simulink model "gm_sd_filter_tb"  (R2022b)
settings: Solver=VariableStepAuto  StartTime=0.0  StopTime=t_stop  RelTol=1e-3
undefined symbols (not defined in the file or in its folder): bitwidths, ts
settings Model: Creator=Legion  LastModifiedBy=qaztr
settings SolverCC: AlgebraicLoopSolver=TrustRegion
settings OptimizationCC: BlockReduction=off  ConditionallyExecuteInputs=off
settings DebuggingCC: InheritedTsInSrcMsg=none  UnconnectedInputMsg=warning  UnconnectedOutputMsg=warning  UnconnectedLineMsg=warning  SFMachineParentedDataDiag=warning
settings ModelReferenceCC: EnableRefExpFcnMdlSchedulingChecks=on
settings RTWCC: DLArmComputeVersion=19.05

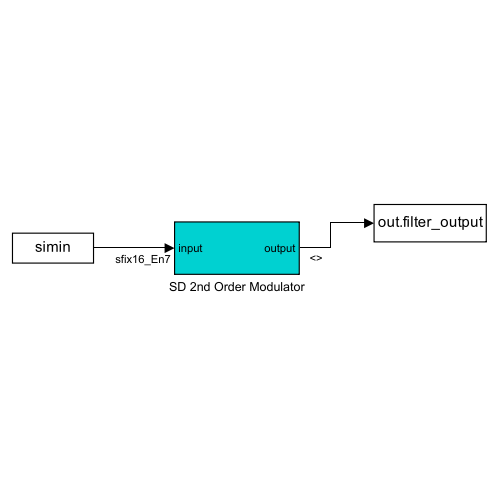
[thumbnail: Simulink's stored preview of the top-level diagram]
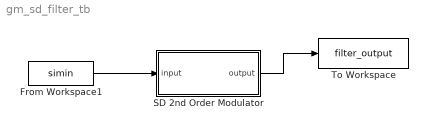
== system gm_sd_filter_tb ==
  From Workspace1 : FromWorkspace  VariableName=simin  SampleTime=ts  Interpolate=off  OutputAfterFinalValue=Holding final value
  SD 2nd Order Modulator : Subsystem
  To Workspace : ToWorkspace  VariableName=filter_output  SaveFormat=Structure With Time  SampleTime=-1
  wires:
  From Workspace1/1 -> SD 2nd Order Modulator/1(input)
  SD 2nd Order Modulator/1(output) -> To Workspace/1

== system gm_sd_filter_tb/SD 2nd Order Modulator ==
  input : Inport  OutDataTypeStr=fixdt(1, 16, 7)  PortDimensions=1  SampleTime=8.85770975056689e-08
  SD 2nd Order Modulator : Subsystem
  SD 2nd Order Modulator1 : Subsystem
  SD Filter : Subsystem
  output : Outport  SampleTime=8.85770975056689e-08
  wires:
  input/1 -> SD 2nd Order Modulator1/1(in)
  SD 2nd Order Modulator/1(out) -> output/1, SD Filter/2(feedback)
  SD 2nd Order Modulator1/1(out) -> SD Filter/1(input)
  SD Filter/1(output) -> SD 2nd Order Modulator/1(in)

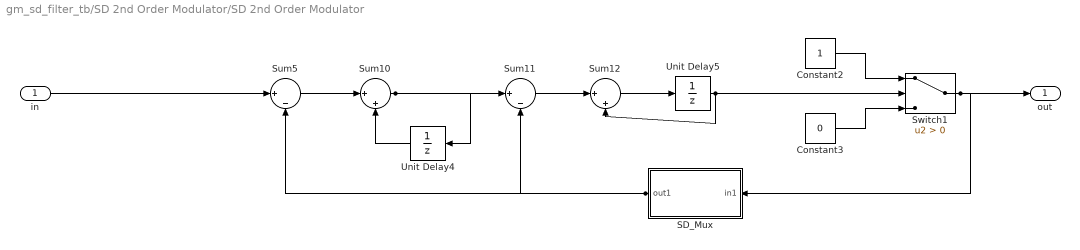
== system gm_sd_filter_tb/SD 2nd Order Modulator/SD 2nd Order Modulator ==
  in : Inport  OutDataTypeStr=fixdt(1, 47, 22)  PortDimensions=1  SampleTime=8.85770975056689e-08
  Constant2 : Constant  OutDataTypeStr=boolean
  Constant3 : Constant  Value=0  OutDataTypeStr=boolean
  SD_Mux : Subsystem  mask{a=fi(0,1,16,7,"hex","0080"), Parameter2=fixdt(1,32,23)}
      mask prompts: a "Amp"; Parameter2 "Data Type"
  Sum10 : Sum  Inputs=||+|+  OutDataTypeStr=Inherit: Same as accumulator
  Sum11 : Sum  Inputs=||+|-  OutDataTypeStr=Inherit: Same as accumulator
  Sum12 : Sum  Inputs=||+|+  OutDataTypeStr=Inherit: Same as accumulator
  Sum5 : Sum  Inputs=||+|-  OutDataTypeStr=Inherit: Same as accumulator
  Switch1 : Switch  Criteria=u2 > Threshold  SaturateOnIntegerOverflow=off  InputSameDT=off
  Unit Delay4 : UnitDelay  SampleTime=-1  HasFrameUpgradeWarning=on
  Unit Delay5 : UnitDelay  SampleTime=-1  HasFrameUpgradeWarning=on
  out : Outport  SampleTime=8.85770975056689e-08
  wires:
  in/1 -> Sum5/1
  Constant2/1 -> Switch1/1
  Constant3/1 -> Switch1/3
  SD_Mux/1(out1) -> Sum5/2, Sum11/2
  Sum10/1 -> Sum11/1, Unit Delay4/1
  Sum11/1 -> Sum12/1
  Sum12/1 -> Unit Delay5/1
  Sum5/1 -> Sum10/1
  Switch1/1 -> SD_Mux/1(in1), out/1
  Unit Delay4/1 -> Sum10/2
  Unit Delay5/1 -> Switch1/2, Sum12/2

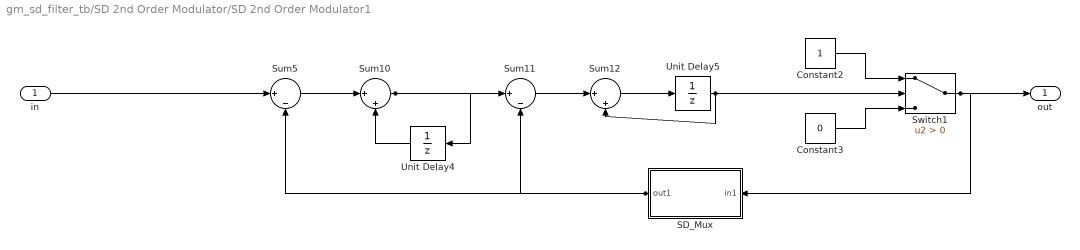
== system gm_sd_filter_tb/SD 2nd Order Modulator/SD 2nd Order Modulator1 ==
  in : Inport  OutDataTypeStr=fixdt(1, 16, 7)  PortDimensions=1  SampleTime=8.85770975056689e-08
  Constant2 : Constant  OutDataTypeStr=boolean
  Constant3 : Constant  Value=0  OutDataTypeStr=boolean
  SD_Mux : Subsystem  mask{a=fi(0,1,16,7,"hex","0080"), Parameter2=fixdt(1,32,23)}
      mask prompts: a "Amp"; Parameter2 "Data Type"
  Sum10 : Sum  Inputs=||+|+  OutDataTypeStr=Inherit: Same as accumulator
  Sum11 : Sum  Inputs=||+|-  OutDataTypeStr=Inherit: Same as accumulator
  Sum12 : Sum  Inputs=||+|+  OutDataTypeStr=Inherit: Same as accumulator
  Sum5 : Sum  Inputs=||+|-  OutDataTypeStr=Inherit: Same as accumulator
  Switch1 : Switch  Criteria=u2 > Threshold  SaturateOnIntegerOverflow=off  InputSameDT=off
  Unit Delay4 : UnitDelay  SampleTime=-1  HasFrameUpgradeWarning=on
  Unit Delay5 : UnitDelay  SampleTime=-1  HasFrameUpgradeWarning=on
  out : Outport  SampleTime=8.85770975056689e-08
  wires:
  in/1 -> Sum5/1
  Constant2/1 -> Switch1/1
  Constant3/1 -> Switch1/3
  SD_Mux/1(out1) -> Sum5/2, Sum11/2
  Sum10/1 -> Sum11/1, Unit Delay4/1
  Sum11/1 -> Sum12/1
  Sum12/1 -> Unit Delay5/1
  Sum5/1 -> Sum10/1
  Switch1/1 -> SD_Mux/1(in1), out/1
  Unit Delay4/1 -> Sum10/2
  Unit Delay5/1 -> Switch1/2, Sum12/2

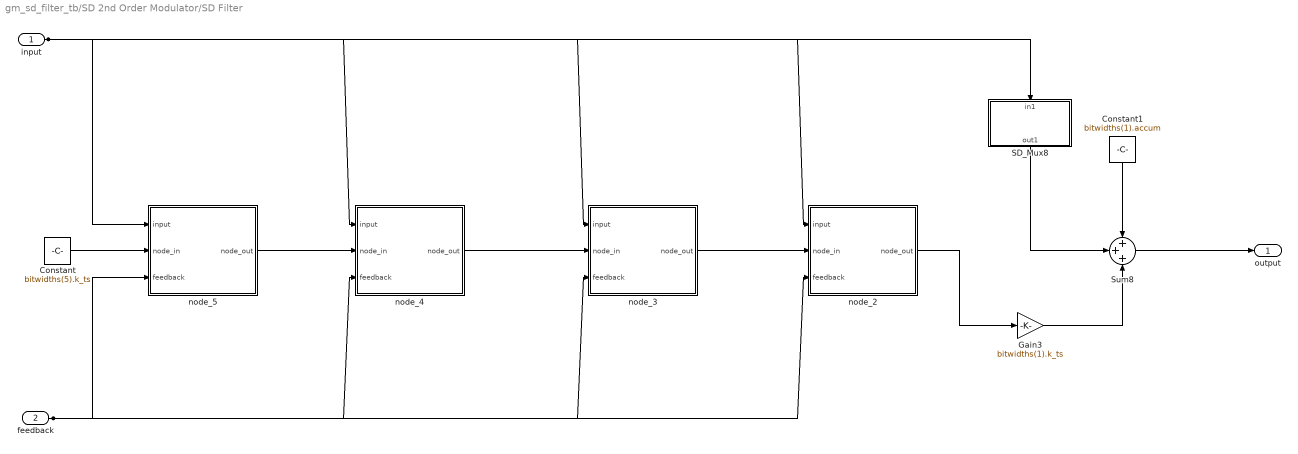
== system gm_sd_filter_tb/SD 2nd Order Modulator/SD Filter ==
  input : Inport  OutDataTypeStr=boolean  PortDimensions=1  SampleTime=8.85770975056689e-08
  feedback : Inport  Port=2  OutDataTypeStr=boolean  PortDimensions=1  SampleTime=8.85770975056689e-08
  Constant : Constant  Value=bitwidths(5).k_ts
  Constant1 : Constant  Value=bitwidths(1).accum
  Gain3 : Gain  Gain=bitwidths(1).k_ts  RndMeth=Round
  SD_Mux8 : Subsystem  mask{a=fi(0,1,24,22,"hex","001062"), Parameter2=Inherit: Inherit via internal rule}
      mask prompts: a "Amp"; Parameter2 "Data Type"
  Sum8 : Sum  Inputs=+++  OutDataTypeStr=Inherit: Same as accumulator
  node_2 : Subsystem  mask{Parameter1=fi(0,1,21,8,"hex","064305"), Parameter2=fi(0,1,21,8,"hex","00000c"), Parameter3=fi(0,1,12,11,"hex","001"), Parameter4=fi(0,1,33,8,"hex","000000000")}
      mask prompts: Parameter1 "alpha"; Parameter2 "beta"; Parameter3 "k"; Parameter4 "Accumulator"
  node_3 : Subsystem  mask{Parameter1=fi(0,1,25,8,"hex","04b7082"), Parameter2=fi(0,1,25,8,"hex","000adcd"), Parameter3=fi(0,1,12,11,"hex","001"), Parameter4=fi(0,1,33,8,"hex","000000000")}
      mask prompts: Parameter1 "alpha"; Parameter2 "beta"; Parameter3 "k"; Parameter4 "Accumulator"
  node_4 : Subsystem  mask{Parameter1=fi(0,1,21,8,"hex","07523c"), Parameter2=fi(0,1,21,8,"hex","0022af"), Parameter3=fi(0,1,12,11,"hex","001"), Parameter4=fi(0,1,33,8,"hex","000000000")}
      mask prompts: Parameter1 "alpha"; Parameter2 "beta"; Parameter3 "k"; Parameter4 "Accumulator"
  node_5 : Subsystem  mask{Parameter1=fi(0,1,16,0,"hex","2bbf"), Parameter2=fi(0,1,16,0,"hex","000b"), Parameter3=fi(0,1,2,1,"hex","0"), Parameter4=fi(0,1,25,0,"hex","0000000")}
      mask prompts: Parameter1 "alpha"; Parameter2 "beta"; Parameter3 "k"; Parameter4 "Accumulator"
  output : Outport  SampleTime=8.85770975056689e-08
  wires:
  input/1 -> node_5/1(input), node_4/1(input), node_3/1(input), node_2/1(input), SD_Mux8/1(in1)
  feedback/1 -> node_5/3(feedback), node_4/3(feedback), node_2/3(feedback), node_3/3(feedback)
  Constant/1 -> node_5/2(node_in)
  Constant1/1 -> Sum8/1
  Gain3/1 -> Sum8/3
  SD_Mux8/1(out1) -> Sum8/2
  Sum8/1 -> output/1
  node_2/1(node_out) -> Gain3/1
  node_3/1(node_out) -> node_2/2(node_in)
  node_4/1(node_out) -> node_3/2(node_in)
  node_5/1(node_out) -> node_4/2(node_in)

== system gm_sd_filter_tb/SD 2nd Order Modulator/SD 2nd Order Modulator/SD_Mux ==
  in1 : Inport  OutDataTypeStr=boolean  PortDimensions=1  SampleTime=8.85770975056689e-08
  Constant2 : Constant  Value=a
  Constant3 : Constant  Value=-a
  Switch1 : Switch  Criteria=u2 > Threshold  SaturateOnIntegerOverflow=off  InputSameDT=off
  out1 : Outport  SampleTime=8.85770975056689e-08
  wires:
  in1/1 -> Switch1/2
  Constant2/1 -> Switch1/1
  Constant3/1 -> Switch1/3
  Switch1/1 -> out1/1

== system gm_sd_filter_tb/SD 2nd Order Modulator/SD 2nd Order Modulator1/SD_Mux ==
  in1 : Inport  OutDataTypeStr=boolean  PortDimensions=1  SampleTime=8.85770975056689e-08
  Constant2 : Constant  Value=a
  Constant3 : Constant  Value=-a
  Switch1 : Switch  Criteria=u2 > Threshold  SaturateOnIntegerOverflow=off  InputSameDT=off
  out1 : Outport  SampleTime=8.85770975056689e-08
  wires:
  in1/1 -> Switch1/2
  Constant2/1 -> Switch1/1
  Constant3/1 -> Switch1/3
  Switch1/1 -> out1/1

== system gm_sd_filter_tb/SD 2nd Order Modulator/SD Filter/SD_Mux8 ==
  in1 : Inport  OutDataTypeStr=boolean  PortDimensions=1  SampleTime=8.85770975056689e-08
  Constant2 : Constant  Value=a
  Constant3 : Constant  Value=-a
  Switch1 : Switch  Criteria=u2 > Threshold  SaturateOnIntegerOverflow=off  InputSameDT=off
  out1 : Outport  SampleTime=8.85770975056689e-08
  wires:
  in1/1 -> Switch1/2
  Constant2/1 -> Switch1/1
  Constant3/1 -> Switch1/3
  Switch1/1 -> out1/1

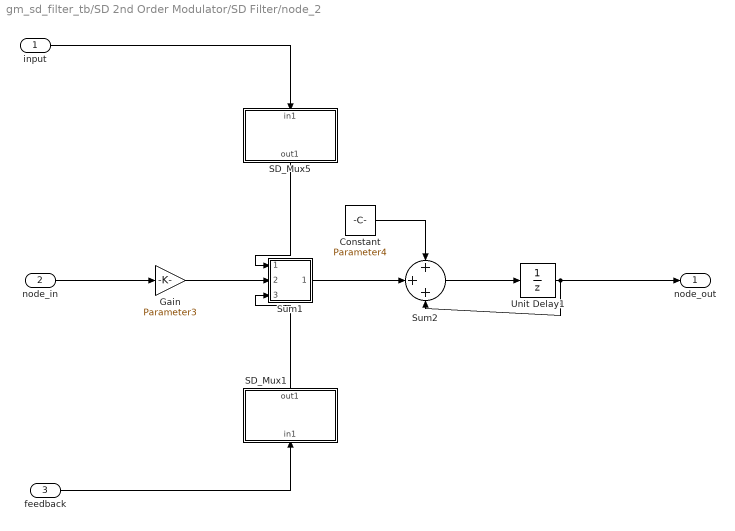
== system gm_sd_filter_tb/SD 2nd Order Modulator/SD Filter/node_2 ==
  input : Inport  OutDataTypeStr=boolean  PortDimensions=1  SampleTime=8.85770975056689e-08
  node_in : Inport  Port=2  OutDataTypeStr=fixdt(1, 33, 8)  PortDimensions=1  SampleTime=8.85770975056689e-08
  feedback : Inport  Port=3  OutDataTypeStr=boolean  PortDimensions=1  SampleTime=8.85770975056689e-08
  Constant : Constant  Value=Parameter4
  Gain : Gain  Gain=Parameter3  RndMeth=Round
  SD_Mux1 : Subsystem  mask{a=fi(0,1,21,8,"hex","064305"), Parameter2=Inherit: Inherit via internal rule}
      mask prompts: a "Amp"; Parameter2 "Data Type"
  SD_Mux5 : Subsystem  mask{a=fi(0,1,21,8,"hex","00000c"), Parameter2=Inherit: Inherit via internal rule}
      mask prompts: a "Amp"; Parameter2 "Data Type"
  Sum1 : Subsystem
  Sum2 : Sum  Inputs=+++  OutDataTypeStr=Inherit: Same as accumulator
  Unit Delay1 : UnitDelay  SampleTime=-1  HasFrameUpgradeWarning=on
  node_out : Outport  SampleTime=8.85770975056689e-08
  wires:
  input/1 -> SD_Mux5/1(in1)
  node_in/1 -> Gain/1
  feedback/1 -> SD_Mux1/1(in1)
  Constant/1 -> Sum2/1
  Gain/1 -> Sum1/2(In2)
  SD_Mux1/1(out1) -> Sum1/3(In3)
  SD_Mux5/1(out1) -> Sum1/1(In1)
  Sum1/1(Out1) -> Sum2/2
  Sum2/1 -> Unit Delay1/1
  Unit Delay1/1 -> Sum2/3, node_out/1

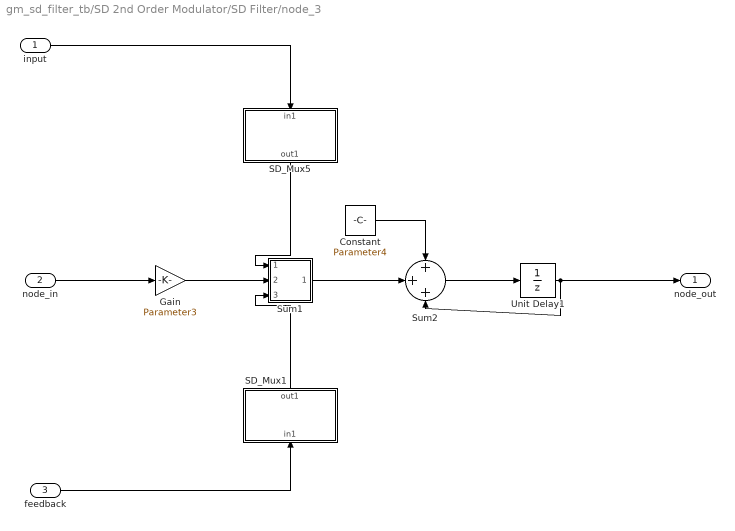
== system gm_sd_filter_tb/SD 2nd Order Modulator/SD Filter/node_3 ==
  input : Inport  OutDataTypeStr=boolean  PortDimensions=1  SampleTime=8.85770975056689e-08
  node_in : Inport  Port=2  OutDataTypeStr=fixdt(1, 33, 8)  PortDimensions=1  SampleTime=8.85770975056689e-08
  feedback : Inport  Port=3  OutDataTypeStr=boolean  PortDimensions=1  SampleTime=8.85770975056689e-08
  Constant : Constant  Value=Parameter4
  Gain : Gain  Gain=Parameter3  RndMeth=Round
  SD_Mux1 : Subsystem  mask{a=fi(0,1,25,8,"hex","04b7082"), Parameter2=Inherit: Inherit via internal rule}
      mask prompts: a "Amp"; Parameter2 "Data Type"
  SD_Mux5 : Subsystem  mask{a=fi(0,1,25,8,"hex","000adcd"), Parameter2=Inherit: Inherit via internal rule}
      mask prompts: a "Amp"; Parameter2 "Data Type"
  Sum1 : Subsystem
  Sum2 : Sum  Inputs=+++  OutDataTypeStr=Inherit: Same as accumulator
  Unit Delay1 : UnitDelay  SampleTime=-1  HasFrameUpgradeWarning=on
  node_out : Outport  SampleTime=8.85770975056689e-08
  wires:
  input/1 -> SD_Mux5/1(in1)
  node_in/1 -> Gain/1
  feedback/1 -> SD_Mux1/1(in1)
  Constant/1 -> Sum2/1
  Gain/1 -> Sum1/2(In2)
  SD_Mux1/1(out1) -> Sum1/3(In3)
  SD_Mux5/1(out1) -> Sum1/1(In1)
  Sum1/1(Out1) -> Sum2/2
  Sum2/1 -> Unit Delay1/1
  Unit Delay1/1 -> Sum2/3, node_out/1

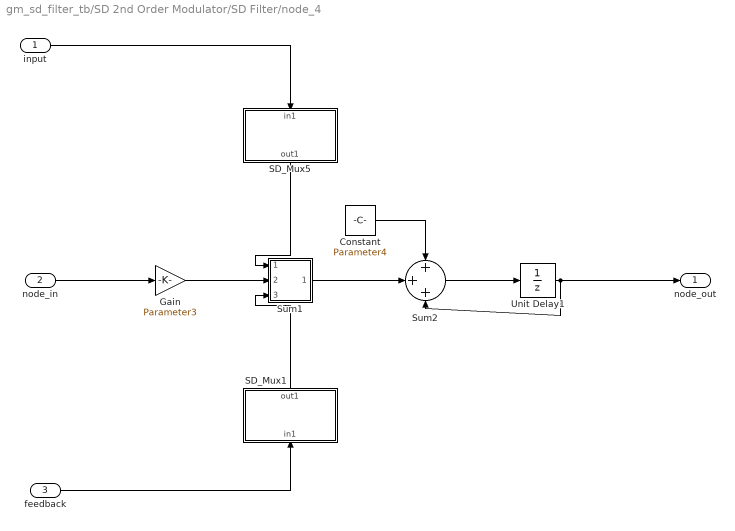
== system gm_sd_filter_tb/SD 2nd Order Modulator/SD Filter/node_4 ==
  input : Inport  OutDataTypeStr=boolean  PortDimensions=1  SampleTime=8.85770975056689e-08
  node_in : Inport  Port=2  OutDataTypeStr=fixdt(1, 25, 0)  PortDimensions=1  SampleTime=8.85770975056689e-08
  feedback : Inport  Port=3  OutDataTypeStr=boolean  PortDimensions=1  SampleTime=8.85770975056689e-08
  Constant : Constant  Value=Parameter4
  Gain : Gain  Gain=Parameter3  RndMeth=Round
  SD_Mux1 : Subsystem  mask{a=fi(0,1,21,8,"hex","07523c"), Parameter2=Inherit: Inherit via internal rule}
      mask prompts: a "Amp"; Parameter2 "Data Type"
  SD_Mux5 : Subsystem  mask{a=fi(0,1,21,8,"hex","0022af"), Parameter2=Inherit: Inherit via internal rule}
      mask prompts: a "Amp"; Parameter2 "Data Type"
  Sum1 : Subsystem
  Sum2 : Sum  Inputs=+++  OutDataTypeStr=Inherit: Same as accumulator
  Unit Delay1 : UnitDelay  SampleTime=-1  HasFrameUpgradeWarning=on
  node_out : Outport  SampleTime=8.85770975056689e-08
  wires:
  input/1 -> SD_Mux5/1(in1)
  node_in/1 -> Gain/1
  feedback/1 -> SD_Mux1/1(in1)
  Constant/1 -> Sum2/1
  Gain/1 -> Sum1/2(In2)
  SD_Mux1/1(out1) -> Sum1/3(In3)
  SD_Mux5/1(out1) -> Sum1/1(In1)
  Sum1/1(Out1) -> Sum2/2
  Sum2/1 -> Unit Delay1/1
  Unit Delay1/1 -> Sum2/3, node_out/1

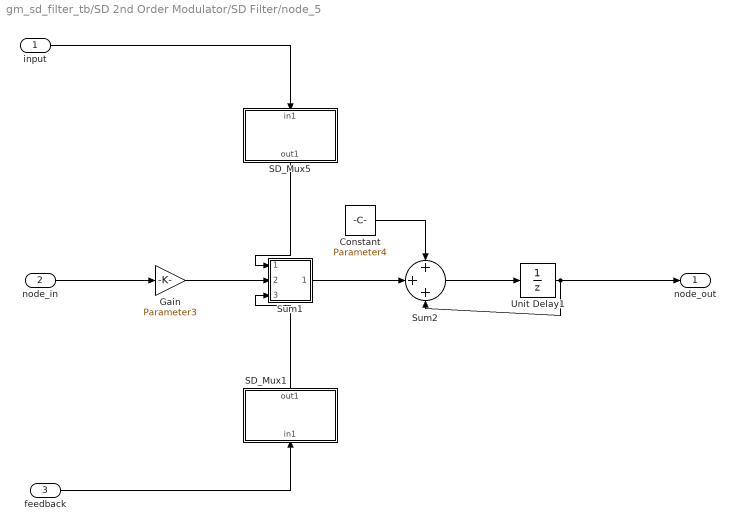
== system gm_sd_filter_tb/SD 2nd Order Modulator/SD Filter/node_5 ==
  input : Inport  OutDataTypeStr=boolean  PortDimensions=1  SampleTime=8.85770975056689e-08
  node_in : Inport  Port=2  OutDataTypeStr=fixdt(1, 2, 1)  PortDimensions=1
  feedback : Inport  Port=3  OutDataTypeStr=boolean  PortDimensions=1  SampleTime=8.85770975056689e-08
  Constant : Constant  Value=Parameter4
  Gain : Gain  Gain=Parameter3  RndMeth=Round
  SD_Mux1 : Subsystem  mask{a=fi(0,1,16,0,"hex","2bbf"), Parameter2=Inherit: Inherit via internal rule}
      mask prompts: a "Amp"; Parameter2 "Data Type"
  SD_Mux5 : Subsystem  mask{a=fi(0,1,16,0,"hex","000b"), Parameter2=Inherit: Inherit via internal rule}
      mask prompts: a "Amp"; Parameter2 "Data Type"
  Sum1 : Subsystem
  Sum2 : Sum  Inputs=+++  OutDataTypeStr=Inherit: Same as accumulator
  Unit Delay1 : UnitDelay  SampleTime=-1  HasFrameUpgradeWarning=on
  node_out : Outport  SampleTime=8.85770975056689e-08
  wires:
  input/1 -> SD_Mux5/1(in1)
  node_in/1 -> Gain/1
  feedback/1 -> SD_Mux1/1(in1)
  Constant/1 -> Sum2/1
  Gain/1 -> Sum1/2(In2)
  SD_Mux1/1(out1) -> Sum1/3(In3)
  SD_Mux5/1(out1) -> Sum1/1(In1)
  Sum1/1(Out1) -> Sum2/2
  Sum2/1 -> Unit Delay1/1
  Unit Delay1/1 -> Sum2/3, node_out/1

== system gm_sd_filter_tb/SD 2nd Order Modulator/SD Filter/node_2/SD_Mux1 ==
  in1 : Inport  OutDataTypeStr=boolean  PortDimensions=1  SampleTime=8.85770975056689e-08
  Constant2 : Constant  Value=a
  Constant3 : Constant  Value=-a
  Switch1 : Switch  Criteria=u2 > Threshold  SaturateOnIntegerOverflow=off  InputSameDT=off
  out1 : Outport  SampleTime=8.85770975056689e-08
  wires:
  in1/1 -> Switch1/2
  Constant2/1 -> Switch1/1
  Constant3/1 -> Switch1/3
  Switch1/1 -> out1/1

== system gm_sd_filter_tb/SD 2nd Order Modulator/SD Filter/node_2/SD_Mux5 ==
  in1 : Inport  OutDataTypeStr=boolean  PortDimensions=1  SampleTime=8.85770975056689e-08
  Constant2 : Constant  Value=a
  Constant3 : Constant  Value=-a
  Switch1 : Switch  Criteria=u2 > Threshold  SaturateOnIntegerOverflow=off  InputSameDT=off
  out1 : Outport  SampleTime=8.85770975056689e-08
  wires:
  in1/1 -> Switch1/2
  Constant2/1 -> Switch1/1
  Constant3/1 -> Switch1/3
  Switch1/1 -> out1/1

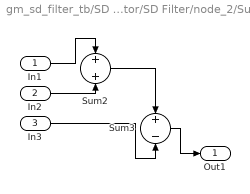
== system gm_sd_filter_tb/SD 2nd Order Modulator/SD Filter/node_2/Sum1 ==
  In1 : Inport  OutDataTypeStr=fixdt(1,21,8)
  In2 : Inport  Port=2  OutDataTypeStr=fixdt(1,66,50)
  In3 : Inport  Port=3  OutDataTypeStr=fixdt(1,21,8)
  Sum2 : Sum  AccumDataTypeStr=fixdt(1,21,8)  OutDataTypeStr=fixdt(1,21,8)
  Sum3 : Sum  Inputs=+-  AccumDataTypeStr=fixdt(1,21,8)  OutDataTypeStr=fixdt(1,21,8)
  Out1 : Outport
  wires:
  In1/1 -> Sum2/1
  In2/1 -> Sum2/2
  Sum2/1 -> Sum3/1
  In3/1 -> Sum3/2
  Sum3/1 -> Out1/1

== system gm_sd_filter_tb/SD 2nd Order Modulator/SD Filter/node_3/SD_Mux1 ==
  in1 : Inport  OutDataTypeStr=boolean  PortDimensions=1  SampleTime=8.85770975056689e-08
  Constant2 : Constant  Value=a
  Constant3 : Constant  Value=-a
  Switch1 : Switch  Criteria=u2 > Threshold  SaturateOnIntegerOverflow=off  InputSameDT=off
  out1 : Outport  SampleTime=8.85770975056689e-08
  wires:
  in1/1 -> Switch1/2
  Constant2/1 -> Switch1/1
  Constant3/1 -> Switch1/3
  Switch1/1 -> out1/1

== system gm_sd_filter_tb/SD 2nd Order Modulator/SD Filter/node_3/SD_Mux5 ==
  in1 : Inport  OutDataTypeStr=boolean  PortDimensions=1  SampleTime=8.85770975056689e-08
  Constant2 : Constant  Value=a
  Constant3 : Constant  Value=-a
  Switch1 : Switch  Criteria=u2 > Threshold  SaturateOnIntegerOverflow=off  InputSameDT=off
  out1 : Outport  SampleTime=8.85770975056689e-08
  wires:
  in1/1 -> Switch1/2
  Constant2/1 -> Switch1/1
  Constant3/1 -> Switch1/3
  Switch1/1 -> out1/1

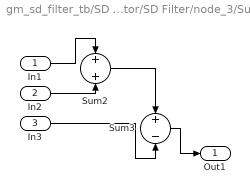
== system gm_sd_filter_tb/SD 2nd Order Modulator/SD Filter/node_3/Sum1 ==
  In1 : Inport  OutDataTypeStr=fixdt(1,25,8)
  In2 : Inport  Port=2  OutDataTypeStr=fixdt(1,66,50)
  In3 : Inport  Port=3  OutDataTypeStr=fixdt(1,25,8)
  Sum2 : Sum  AccumDataTypeStr=fixdt(1,25,8)  OutDataTypeStr=fixdt(1,25,8)
  Sum3 : Sum  Inputs=+-  AccumDataTypeStr=fixdt(1,25,8)  OutDataTypeStr=fixdt(1,25,8)
  Out1 : Outport
  wires:
  In1/1 -> Sum2/1
  In2/1 -> Sum2/2
  Sum2/1 -> Sum3/1
  In3/1 -> Sum3/2
  Sum3/1 -> Out1/1

== system gm_sd_filter_tb/SD 2nd Order Modulator/SD Filter/node_4/SD_Mux1 ==
  in1 : Inport  OutDataTypeStr=boolean  PortDimensions=1  SampleTime=8.85770975056689e-08
  Constant2 : Constant  Value=a
  Constant3 : Constant  Value=-a
  Switch1 : Switch  Criteria=u2 > Threshold  SaturateOnIntegerOverflow=off  InputSameDT=off
  out1 : Outport  SampleTime=8.85770975056689e-08
  wires:
  in1/1 -> Switch1/2
  Constant2/1 -> Switch1/1
  Constant3/1 -> Switch1/3
  Switch1/1 -> out1/1

== system gm_sd_filter_tb/SD 2nd Order Modulator/SD Filter/node_4/SD_Mux5 ==
  in1 : Inport  OutDataTypeStr=boolean  PortDimensions=1  SampleTime=8.85770975056689e-08
  Constant2 : Constant  Value=a
  Constant3 : Constant  Value=-a
  Switch1 : Switch  Criteria=u2 > Threshold  SaturateOnIntegerOverflow=off  InputSameDT=off
  out1 : Outport  SampleTime=8.85770975056689e-08
  wires:
  in1/1 -> Switch1/2
  Constant2/1 -> Switch1/1
  Constant3/1 -> Switch1/3
  Switch1/1 -> out1/1

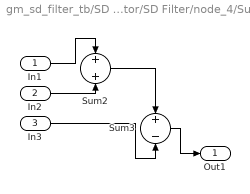
== system gm_sd_filter_tb/SD 2nd Order Modulator/SD Filter/node_4/Sum1 ==
  In1 : Inport  OutDataTypeStr=fixdt(1,21,8)
  In2 : Inport  Port=2  OutDataTypeStr=fixdt(1,50,34)
  In3 : Inport  Port=3  OutDataTypeStr=fixdt(1,21,8)
  Sum2 : Sum  AccumDataTypeStr=fixdt(1,21,8)  OutDataTypeStr=fixdt(1,21,8)
  Sum3 : Sum  Inputs=+-  AccumDataTypeStr=fixdt(1,21,8)  OutDataTypeStr=fixdt(1,21,8)
  Out1 : Outport
  wires:
  In1/1 -> Sum2/1
  In2/1 -> Sum2/2
  Sum2/1 -> Sum3/1
  In3/1 -> Sum3/2
  Sum3/1 -> Out1/1

== system gm_sd_filter_tb/SD 2nd Order Modulator/SD Filter/node_5/SD_Mux1 ==
  in1 : Inport  OutDataTypeStr=boolean  PortDimensions=1  SampleTime=8.85770975056689e-08
  Constant2 : Constant  Value=a
  Constant3 : Constant  Value=-a
  Switch1 : Switch  Criteria=u2 > Threshold  SaturateOnIntegerOverflow=off  InputSameDT=off
  out1 : Outport  SampleTime=8.85770975056689e-08
  wires:
  in1/1 -> Switch1/2
  Constant2/1 -> Switch1/1
  Constant3/1 -> Switch1/3
  Switch1/1 -> out1/1

== system gm_sd_filter_tb/SD 2nd Order Modulator/SD Filter/node_5/SD_Mux5 ==
  in1 : Inport  OutDataTypeStr=boolean  PortDimensions=1  SampleTime=8.85770975056689e-08
  Constant2 : Constant  Value=a
  Constant3 : Constant  Value=-a
  Switch1 : Switch  Criteria=u2 > Threshold  SaturateOnIntegerOverflow=off  InputSameDT=off
  out1 : Outport  SampleTime=8.85770975056689e-08
  wires:
  in1/1 -> Switch1/2
  Constant2/1 -> Switch1/1
  Constant3/1 -> Switch1/3
  Switch1/1 -> out1/1

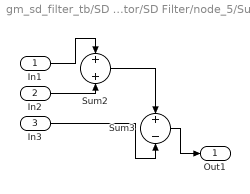
== system gm_sd_filter_tb/SD 2nd Order Modulator/SD Filter/node_5/Sum1 ==
  In1 : Inport  OutDataTypeStr=fixdt(1,16,0)
  In2 : Inport  Port=2  OutDataTypeStr=fixdt(1,8,1001)
  In3 : Inport  Port=3  OutDataTypeStr=fixdt(1,16,0)
  Sum2 : Sum  AccumDataTypeStr=fixdt(1,16,0)  OutDataTypeStr=fixdt(1,16,0)
  Sum3 : Sum  Inputs=+-  AccumDataTypeStr=fixdt(1,16,0)  OutDataTypeStr=fixdt(1,16,0)
  Out1 : Outport
  wires:
  In1/1 -> Sum2/1
  In2/1 -> Sum2/2
  Sum2/1 -> Sum3/1
  In3/1 -> Sum3/2
  Sum3/1 -> Out1/1
